simulink model "battery_finite_state_machine"  (R2022b)
settings: Solver=FixedStepDiscrete  StartTime=0.0  StopTime=10.0  FixedStep=0.1  RelTol=1e-3  EnableMultiTasking=on
settings Model: Creator=jlosi  LastModifiedBy=jlosi
settings SolverCC: AlgebraicLoopSolver=TrustRegion  AutoInsertRateTranBlk=on
settings DataIOCC: LimitDataPoints=on
settings OptimizationCC: LifeSpan=inf
settings DebuggingCC: UnconnectedInputMsg=warning  UnconnectedOutputMsg=warning  UnconnectedLineMsg=warning  AllowSymbolicDim=off  SFUnexpectedBacktrackingDiag=warning  SFNoUnconditionalDefaultTransitionDiag=warning  SFExecutionAtInitializationDiag=none  ArithmeticOperatorsInVariantConditions=warning
settings ModelReferenceCC: EnableRefExpFcnMdlSchedulingChecks=on
settings SFSimCC: SimUseLocalCustomCode=off  CustomCodeUndefinedFunction=UseInterfaceOnly
settings RTWCC: RTWUseLocalCustomCode=off  DLArmComputeVersion=19.05
settings CodeAppCC: StateflowObjectComments=on
settings GRTTargetCC: TargetLangStandard=C89/C90 (ANSI)
settings ConfigComp: CovMetricSettings=dw  CovSaveCumulativeToWorkspaceVar=on  CovSaveSingleToWorkspaceVar=on  CovExternalEMLEnable=off  CovSFcnEnable=off

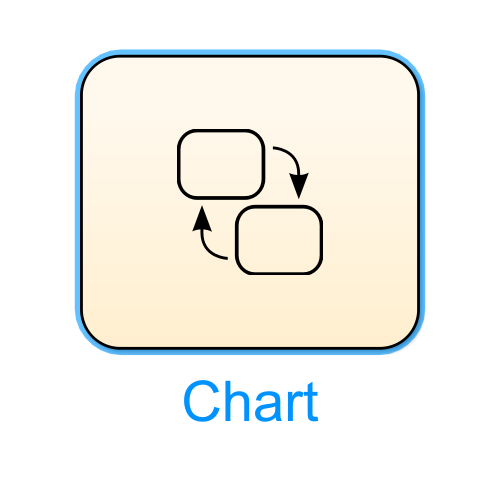
[thumbnail: Simulink's stored preview of the top-level diagram]
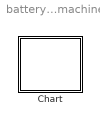
== system battery_finite_state_machine ==
  Chart : Stateflow chart  TreatAsAtomicUnit=on

== stateflow chart battery_finite_state_machine/Chart ==
  state BATTERY_OK_STANBY
  note: NOTES: verify if timing for starting is correct
      | 10 msec or other
  note: NOTE: the LED as stable RED, should be triggered
      | as soon as we enter the status and keep it as it is
      | during the status or the GPIO pin should be triggered
      | when we exit the status.
      | In the former case, what should we do as the exit condition (?nothing?)
      | If this is considered as a final (exit) status, what heppens when we exit it
  state BATTERY_OK_CPU_READY
    entry,during: setButtonCpuLedRed
  state BATTERY_OK_BOARDS_READY
  state BATTERY_OK_CPU_OFF
    entry,during: setButtonCpuLedRed; setCpuOff;
    exit: setButtonCpuLedRed;
  note: NOTE: EVENT--> User has pushed the button
      | I move from status READY to STARTING iff the user
      | pushes the CPU button
  state BATTERY_CPU_STARTING
    during: setButtonCpuLedFlashingGreen
  state BATTERY_OK_BOARDS_OFF
    during: setButtonBoardsLedRed; setBoardsOff
  state BATTERY_OK_CPU_ON
    entry,during: setButtonCpuLedGreen
  state BATTERY_OK_HSM_RAMPING
  state BATTERY_OK_IN_USE
  state BATTERY_NOK_RESTARTING_CPU
  note: NOTE: In order to make boards or cpu restarting the user
      | must push and hold the button on the back of the robot
      | for 3 seconds. Otherwise we should remain in the previous error
      | status.
      | Thus, theoretically, the behavior of the boards should be as follows:
      | - error -> boards flashing showing error status and motors should be shut down
      | for save them (if error in cpu same behavior)
      | - if we check that the error is not serious, hold and restart the motors/cpu
      | so we reach this status
      | - otherwise we remain in the faulty status with cpu/boards switched off
      |  (from and electronical pov)
  state BATTERY_NOK_RESTARTING_BOARDS
  state BATTERY_NOK_CPU_FAULT
    entry: setEnCpuOff;
    during: setButtonCpuLedFlashingRed;
  state BATTERY_OK_BOARDS_ON
  state BATTERY_NOK_HSM_FAULT
    entry: setEnBoardsOff;
    during: setButtonBoardsLedFlashingRed;
  state BATTERY_NOK_BOARDS_FAULT
    entry: setEnBoardsOff;
    during: setButtonBoardsLedFlashingRed;
  state BATTERY_NOK_BOARDS_LINE_FULL_FAULT
    entry: setEnBoardsOff;
    during: setButtonBoardsLedFlashingRed;
  BATTERY_NOK_RESTARTING_BOARDS -> BATTERY_OK_HSM_RAMPING : [areBoardsAlive]
  (default) -> BATTERY_OK_STANBY
  BATTERY_OK_STANBY -> BATTERY_OK_CPU_READY [order 1] : after(50, msec)
  BATTERY_OK_STANBY -> BATTERY_OK_BOARDS_READY [order 2] : after(50,msec)
  BATTERY_OK_BOARDS_READY -> BATTERY_OK_HSM_RAMPING : [areBoardsAlive]
  BATTERY_OK_CPU_READY -> BATTERY_CPU_STARTING : [isNotYetAlive]
  BATTERY_OK_IN_USE -> BATTERY_OK_CPU_OFF [order 4] : [hasCpuSwitchedOff]
  BATTERY_CPU_STARTING -> BATTERY_OK_CPU_ON : after(500, msec)[isCpuAlive]
  BATTERY_OK_IN_USE -> BATTERY_OK_BOARDS_OFF [order 3] : [haveBoardsSwitchedOff]
  BATTERY_NOK_RESTARTING_CPU -> BATTERY_OK_CPU_ON : [isCpuAlive]
  BATTERY_OK_CPU_ON -> (junction 56)
  BATTERY_OK_HSM_RAMPING -> BATTERY_OK_BOARDS_ON : [isHsmCharged]
  BATTERY_NOK_CPU_FAULT -> BATTERY_NOK_RESTARTING_CPU : [isButtonCpuRestarting]
  BATTERY_OK_IN_USE -> BATTERY_NOK_CPU_FAULT [order 2] : [hasCpuFaulted]
  (junction 56) -> BATTERY_OK_IN_USE : [isCpuAlive && isHsmCharged]
  BATTERY_OK_IN_USE -> (junction 73) [order 1] : [hasHsmFaulted || haveBoardsFaulted]
  (junction 80) -> BATTERY_NOK_RESTARTING_BOARDS
  BATTERY_NOK_HSM_FAULT -> (junction 80) : [isButtonBoardsRestarting]
  BATTERY_NOK_BOARDS_FAULT -> (junction 80) : [isButtonBoardsRestarting]
  BATTERY_OK_BOARDS_ON -> (junction 56)
  (junction 73) -> BATTERY_NOK_HSM_FAULT [order 1] : [hasHsmFaulted]
  (junction 73) -> BATTERY_NOK_BOARDS_LINE_FULL_FAULT [order 3] : [hasHsmFaulted && haveBoardsFaulted]
  (junction 73) -> BATTERY_NOK_BOARDS_FAULT [order 2] : [haveBoardsFaulted]
  data: boardsEnOff function_output; boardsLedFlashRed function_output; boardsOff function_output; boardsLedRed function_output; cpuLedFalshRed function_output; cpuAlive function_output; cpuPinOff function_output; cpuLedGreen function_output; cpuLedRed function_output; bordsAlive function_output; cpuOff function_output; boardsFault function_output; cpuAlive function_output; buttonCpuRestarted function_output; buttonBoardsRestarted function_output; hsmFaultFlag function_output; boardsOFf function_output; hsmCharged function_output; cpuButtonFlashGreen function_output; cpuOff function_output; cpuFaultFlag function_output
  function boardsEnOff = setEnBoardsOff:
    | %#define HSM_EN_OFF        HAL_GPIO_WritePin(HSM_EN, GPIO_PIN_RESET);
    | function boardsEnOff = setEnBoardsOff()
    | 
    |     boardsEnOff = true;
    | 
    | end
  function boardsLedFlashRed = setButtonBoardsLedFlashingRed:
    | function boardsLedFlashRed = setButtonBoardsLedFlashingRed()
    | 
    |     boardsLedFlashRed = true;
    | 
    | end
  function boardsOff = setBoardsOff:
    | function boardsOff = setBoardsOff()
    |     boardsOff = true;
    | end
  function boardsLedRed = setButtonBoardsLedRed:
    | function boardsLedRed = setButtonBoardsLedRed()
    |     boardsLedRed = true;
    | end
  function cpuLedFalshRed = setButtonCpuLedFlashingRed:
    | function cpuLedFalshRed = setButtonCpuLedFlashingRed()
    |     cpuLedFalshRed = true;
    | end
  function cpuAlive = isNotYetAlive:
    | function cpuAlive = isNotYetAlive()
    | 
    |     cpuAlive = false;
    | 
    | end
  function cpuPinOff = setEnCpuOff:
    | %#define EN_V12board_OFF		HAL_GPIO_WritePin(V12board_EN, GPIO_PIN_RESET);
    | function cpuPinOff = setEnCpuOff()
    |     cpuPinOff = true;
    | end
  function cpuLedGreen = setButtonCpuLedGreen:
    | %#define EN_V12board_ON		HAL_GPIO_WritePin(V12board_EN, GPIO_PIN_SET);
    | function cpuLedGreen = setButtonCpuLedGreen()
    |     cpuLedGreen = true;
    | end
  function cpuLedRed = setButtonCpuLedRed:
    | %define PB1_LED_RED       HAL_GPIO_WritePin(CPU_Green, GPIO_PIN_RESET);       HAL_GPIO_WritePin(CPU_Red, GPIO_PIN_SET);
    | function cpuLedRed = setButtonCpuLedRed()
    |     cpuLedRed = true;
    | end
  function bordsAlive = areBoardsAlive:
    | % function should take as input the pointer to bat_bits_array
    | % or the value of the specific bit to check
    | % return a boolean depending on the checked bit
    | function bordsAlive = areBoardsAlive()
    |     bordsAlive = true;
    | end
  function cpuOff = hasCpuSwitchedOff:
    | % #define EN_V12board_OFF		HAL_GPIO_WritePin(V12board_EN, GPIO_PIN_RESET);
    | % #define PB1_LED_RED       HAL_GPIO_WritePin(CPU_Green, GPIO_PIN_RESET);       HAL_GPIO_WritePin(CPU_Red, GPIO_PIN_SET);
    | 
    | function cpuOff = hasCpuSwitchedOff
    |     cpuOff = true;
    | end
  function boardsFault = haveBoardsFaulted:
    | function boardsFault = haveBoardsFaulted()
    |     boardsFault = true;
    | end
  function cpuAlive = isCpuAlive:
    | function cpuAlive = isCpuAlive()
    |     cpuAlive = true;
    | end
  function buttonCpuRestarted = isButtonCpuRestarting:
    | function buttonCpuRestarted = isButtonCpuRestarting()
    |     buttonCpuRestarted = true;
    | end
  function buttonBoardsRestarted = isButtonBoardsRestarting:
    | function buttonBoardsRestarted = isButtonBoardsRestarting
    |     buttonBoardsRestarted = true;
    | end
  function hsmFaultFlag = hasHsmFaulted:
    | function hsmFaultFlag = hasHsmFaulted()
    |     hsmFaultFlag = true;
    | end
  function boardsOFf = haveBoardsSwitchedOff:
    | function boardsOFf = haveBoardsSwitchedOff()
    |     boardsOff = true;
    | end
  function hsmCharged = isHsmCharged:
    | function hsmCharged = isHsmCharged()
    |     hsmCharged = true;
    | end
  function cpuButtonFlashGreen = setButtonCpuLedFlashingGreen:
    | function cpuButtonFlashGreen = setButtonCpuLedFlashingGreen()
    |     cpuButtonFlashGreen = true;
    | end
  function cpuOff = setCpuOff:
    | % #define EN_V12board_OFF		HAL_GPIO_WritePin(V12board_EN, GPIO_PIN_RESET);
    | function cpuOff = setCpuOff()
    |     cpuOff = true;
    | end
  function cpuFaultFlag = hasCpuFaulted:
    | function cpuFaultFlag = hasCpuFaulted()
    |     cpuFaultFlag = true;
    | end
